simulink model "ph_plant_sim"  (Simulink 4.00)
settings: Solver=ode45  StartTime=0.0  StopTime=10.0  RelTol=1e-3
values from neighbouring files (symbols this model uses):
  correcting_pH_level_dynamics = 0.12    [setup_ph_plant.m]
  high_pH = 7.2    [setup_ph_plant.m]
  increase_pH = 0.9    [setup_ph_plant.m]
  low_pH = 6.8    [setup_ph_plant.m]
  max_tank_level = 1    [setup_ph_plant.m]
  no_correction = 0.1    [setup_ph_plant.m]
  normal_level_dynamics = 0.1    [setup_ph_plant.m]
  normal_pH = 7.0    (= 7)    [setup_ph_plant.m]
  reduce_pH = -0.7    [setup_ph_plant.m]
  x0 = [0 7.1]    [setup_ph_plant.m]
libraries: simulink_extras x2, simulink3 x1
settings Model: LastModifiedBy=bsilva

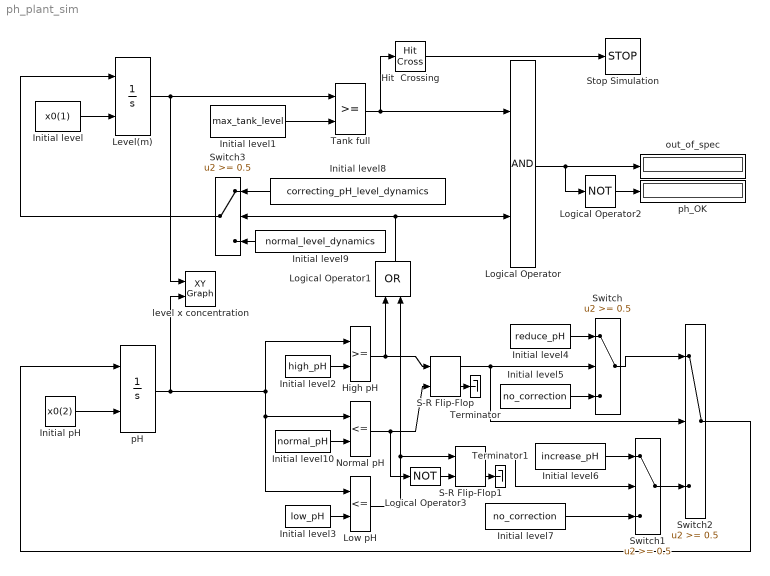
== system ph_plant_sim ==
  High pH : RelationalOperator  Operator=>=
  Hit  Crossing : HitCross  HitCrossingOffset=0.5  HitCrossingDirection=either  ShowOutputPort=on
  Initial level : Constant  Value=x0(1)
  Initial level1 : Constant  Value=max_tank_level
  Initial level10 : Constant  Value=normal_pH
  Initial level2 : Constant  Value=high_pH
  Initial level3 : Constant  Value=low_pH
  Initial level4 : Constant  Value=reduce_pH
  Initial level5 : Constant  Value=no_correction
  Initial level6 : Constant  Value=increase_pH
  Initial level7 : Constant  Value=no_correction
  Initial level8 : Constant  Orientation=left  Value=correcting_pH_level_dynamics
  Initial level9 : Constant  Orientation=left  Value=normal_level_dynamics
  Initial pH : Constant  Value=x0(2)
  Level(m) : Integrator  ExternalReset=none  InitialConditionSource=external  InitialCondition=x0(1)  LimitOutput=off  UpperSaturationLimit=inf  LowerSaturationLimit=-inf  ShowSaturationPort=off  ShowStatePort=off  AbsoluteTolerance=auto
  Logical Operator : Logic  Operator=AND  Inputs=2
  Logical Operator1 : Logic  Orientation=up  Operator=OR  Inputs=2
  Logical Operator2 : Logic  Operator=NOT  Inputs=2
  Logical Operator3 : Logic  Operator=NOT  Inputs=2
  Low pH : RelationalOperator  Operator=<=
  Normal pH : RelationalOperator  Operator=<=
  S-R Flip-Flop : simulink_extras/Flip Flops/S-R Flip-Flop  initial_condition=0
  S-R Flip-Flop1 : simulink_extras/Flip Flops/S-R Flip-Flop  initial_condition=0
  Stop Simulation : Stop
  Switch : Switch  Threshold=0.5
  Switch1 : Switch  Threshold=0.5
  Switch2 : Switch  Threshold=0.5
  Switch3 : Switch  Orientation=left  Threshold=0.5
  Tank full : RelationalOperator  Operator=>=
  Terminator : Terminator
  Terminator1 : Terminator
  level x concentration : simulink3/Sinks/XY Graph  xmin=0  xmax=1  ymin=6.7  ymax=7.3  st=-1
  out_of_spec : Display
      settings: Format=short
  pH : Integrator  ExternalReset=none  InitialConditionSource=external  InitialCondition=0  LimitOutput=off  UpperSaturationLimit=inf  LowerSaturationLimit=-inf  ShowSaturationPort=off  ShowStatePort=off  AbsoluteTolerance=auto
  ph_OK : Display
      settings: Format=short
  wires:
  Initial level/1 -> Level(m)/2
  Initial pH/1 -> pH/2
  Level(m)/1 -> level x concentration/1, Tank full/1
  Initial level1/1 -> Tank full/2
  Tank full/1 -> Hit  Crossing/1, Logical Operator/1
  pH/1 -> level x concentration/2, High pH/1, Low pH/1, Normal pH/1
  Initial level2/1 -> High pH/2
  Initial level3/1 -> Low pH/2
  Initial level5/1 -> Switch/3
  Initial level7/1 -> Switch1/3
  High pH/1 -> Logical Operator1/1, S-R Flip-Flop/1
  Initial level4/1 -> Switch/1
  Initial level6/1 -> Switch1/1
  Low pH/1 -> Logical Operator1/2, S-R Flip-Flop1/1
  Switch1/1 -> Switch2/3
  Switch/1 -> Switch2/1
  Logical Operator1/1 -> Logical Operator/2, Switch3/2
  Logical Operator2/1 -> ph_OK/1
  Logical Operator/1 -> out_of_spec/1, Logical Operator2/1
  Initial level8/1 -> Switch3/1
  Initial level9/1 -> Switch3/3
  Switch2/1 -> pH/1
  Switch3/1 -> Level(m)/1
  Initial level10/1 -> Normal pH/2
  Normal pH/1 -> S-R Flip-Flop/2, Logical Operator3/1
  S-R Flip-Flop/1 -> Switch/2, Switch2/2
  Logical Operator3/1 -> S-R Flip-Flop1/2
  S-R Flip-Flop1/1 -> Switch1/2
  Hit  Crossing/1 -> Stop Simulation/1
  S-R Flip-Flop/2 -> Terminator/1
  S-R Flip-Flop1/2 -> Terminator1/1
